simulink model "lateral_dyn"  (R2020a)
settings: Solver=VariableStepAuto  StartTime=0.0  StopTime=10.0  RelTol=1e-3
settings Model: Creator=User  LastModifiedBy=User

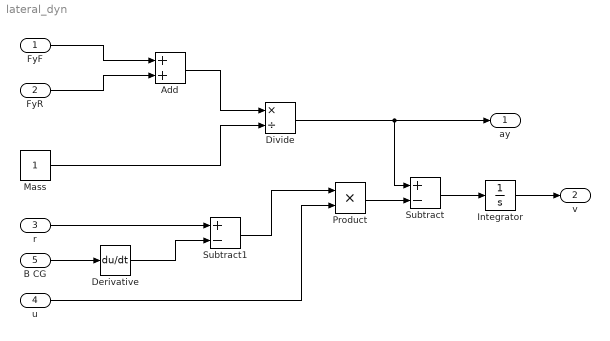
== system lateral_dyn ==
  FyF : Inport
  FyR : Inport  Port=2
  r : Inport  Port=3
  u : Inport  Port=4
  B CG : Inport  Port=5
  Add : Sum
  Derivative : Derivative
  Divide : Product  Inputs=*/
  Integrator : Integrator
  Mass : Constant
  Product : Product
  Subtract : Sum  Inputs=+-
  Subtract1 : Sum  Inputs=+-
  ay : Outport
  v : Outport  Port=2
  wires:
  FyF/1 -> Add/1
  Add/1 -> Divide/1
  Mass/1 -> Divide/2
  Divide/1 -> Subtract/1, ay/1
  Integrator/1 -> v/1
  FyR/1 -> Add/2
  r/1 -> Subtract1/1
  u/1 -> Product/2
  Subtract/1 -> Integrator/1
  Product/1 -> Subtract/2
  B CG/1 -> Derivative/1
  Derivative/1 -> Subtract1/2
  Subtract1/1 -> Product/1
